simulink model "staticQuadricopter_build1"  (R2014b)
settings: Solver=ode45  StartTime=0.0  StopTime=inf  RelTol=1e-3
libraries: LibrarySimulinkSAS x1
settings Model: Creator=DSANTIAGO  LastModifiedBy=DSANTIAGO

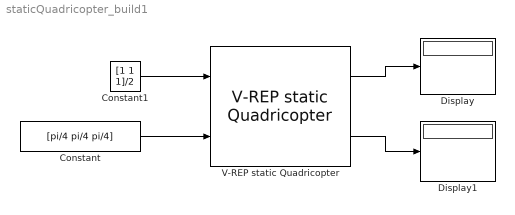
== system staticQuadricopter_build1 ==
  Constant : Constant  Value=[pi/4 pi/4 pi/4]
  Constant1 : Constant  Value=[1 1 1]/2
  Display : Display
  Display1 : Display
  V-REP static Quadricopter : LibrarySimulinkSAS/V-REP static Quadricopter  Id=1
  wires:
  Constant1/1 -> V-REP static Quadricopter/1
  Constant/1 -> V-REP static Quadricopter/2
  V-REP static Quadricopter/1 -> Display/1
  V-REP static Quadricopter/2 -> Display1/1
